simulink library "HX_EN12977"  (Simulink 7.6)
settings: Solver=ode45  StartTime=0.0  StopTime=10.0  RelTol=1e-3
undefined symbols (not defined in the file): dia, height, nodes
libraries: carnot x2
settings Model: Creator=lena.frank  LastModifiedBy=drhf

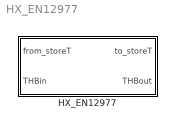
== system HX_EN12977 ==
  HX_EN12977 : Subsystem  mask(heat exchanger for storage, data EN 12977){h_in=0.5, h_out=0, ua0=800, uam=0, uat=0, dplin=100, dpqua=100, nodes=nodes, hgt=height, dia=dia}
      mask prompts: h_in "relative height of inlet"; h_out "relative height of outlet"; ua0 "uac: heat transfer coefficient [W/K /(kg/s) /(°C)]"; uam "uam: massflow dependent heat transfer [-]"; uat "uat: temperature difference dependent heat transfer [-]"; dplin "pressure drop linear in mdot [Pa*s/kg]"; dpqua "pressure drop quadratic in mdot [Pa*s²/kg²]"; nodes "Number of nodes (DO NOT CHANGE)"; hgt "Height vector (DO NOT CHANGE)"; dia "Diameter (DO NOT CHANGE)"
      mask help:
      | The block transforms the incoming THV vector to a vector which the storage interprets as a heat exchanger.
      | Give inlet and outlet as a relative position 0=bottom to 1=top
      | The heat transfer is calculated by:
      | UA = uac * mdot^uam * ((Theatexchanger+Tstorage)/2)^uat
      mask init:
      | in = zeros(nodes,1);    % vector of length nodes
      | up = in;                % vector of length nodes
      | down = in;              % vector of length nodes
      | 
      | h_in = max(0,h_in);     % no nodes below 0
      | h_out = max(0,h_out);   % no nodes below 0
      | 
      | inlet = round(h_in*(nodes-1))+1;    % inlet position
      | outlet = round(h_out*(nodes-1))+1;  % outlet position
      | hgt = (h_out-h_in)*hgt;
      | 
      | in(inlet)=1;
      | 
      | if (h_in < h_out)           % if inlet below outlet
      |     up(inlet:outlet)=1;     % upwards
      | elseif (h_in > h_out)       % else if inlet above outlet
      |     down(outlet:inlet)=1;   % downwards
      | end
      mask Help: web(['file:///' fullfile(path_carnot('help'),'StoragePorts_HeatExchangerModels.html')],'-helpbrowser')
      mask TabNameString: Geometry,Geometry,Heat transfer,Heat transfer,Heat transfer,Pressure drop,Pressure drop,Top mask parameters,Top mask parameters,Top mask parameters
      mask Display: disp('HX EN12977')

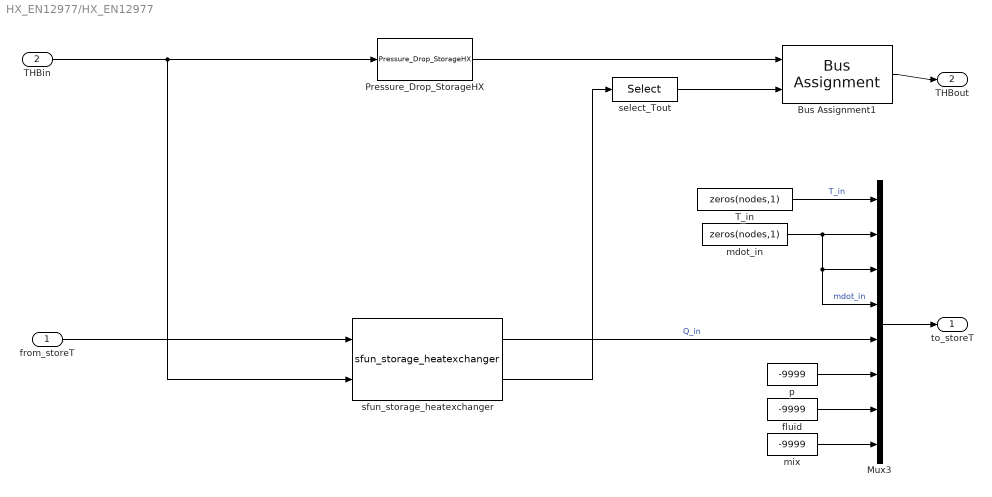
== system HX_EN12977/HX_EN12977 ==
  from_storeT : Inport
  THBin : Inport  Port=2
  Bus Assignment1 : BusAssignment  AssignedSignals=Temperature
  Mux3 : Mux  Inputs=8
  Pressure_Drop_StorageHX : carnot/Basic/Pressure_Drop/Pressure_Drop_StorageHX  SystemSampleTime=-1  dia=dia  hgt=hgt
  T_in : Constant  Value=zeros(nodes,1)
  fluid : Constant  Value=-9999
  mdot_in : Constant  Value=zeros(nodes,1)
  mix : Constant  Value=-9999
  p : Constant  Value=-9999
  select_Tout : Selector  InputPortWidth=nodes  IndexOptions=Index vector (dialog)  Indices=[outlet]  OutputSizes=1
  sfun_storage_heatexchanger : carnot/Basic/Thermal_Models/sfun_storage_heatexchanger  SystemSampleTime=-1  idn=heat transfer data fit EN12977  nodes=nodes  inlet=inlet  outlet=outlet  pp=[ua0, uam, uat, 0,0,0,0]
  to_storeT : Outport  InitialOutput=0
  THBout : Outport  Port=2  InitialOutput=0
  wires:
  Pressure_Drop_StorageHX/1 -> Bus Assignment1/1
  sfun_storage_heatexchanger/2 -> select_Tout/1
  mix/1 -> Mux3/8
  fluid/1 -> Mux3/7
  p/1 -> Mux3/6
  Bus Assignment1/1 -> THBout/1
  sfun_storage_heatexchanger/1 -> Mux3/5  "Q_in"
  T_in/1 -> Mux3/1  "T_in"
  select_Tout/1 -> Bus Assignment1/2
  Mux3/1 -> to_storeT/1
  mdot_in/1 -> Mux3/4, Mux3/3, Mux3/2  "mdot_in"
  THBin/1 -> sfun_storage_heatexchanger/2, Pressure_Drop_StorageHX/1
  from_storeT/1 -> sfun_storage_heatexchanger/1
